simulink model "modele_coque"  (R2025b)
settings: Solver=VariableStepAuto  StartTime=0.0  StopTime=100  RelTol=1e-3
values from neighbouring files (symbols this model uses):
  m = 0.0    (= 0)    [Hulldyn.m]    (also in variables_procom.m = 250000)
  ma = 123434    [variables_procom.m]
  Tc = 0.0    (= 0)    [Hulldyn.m]    (also in variables_procom.m)
settings Model: Creator=leagr  LastModifiedBy=flo

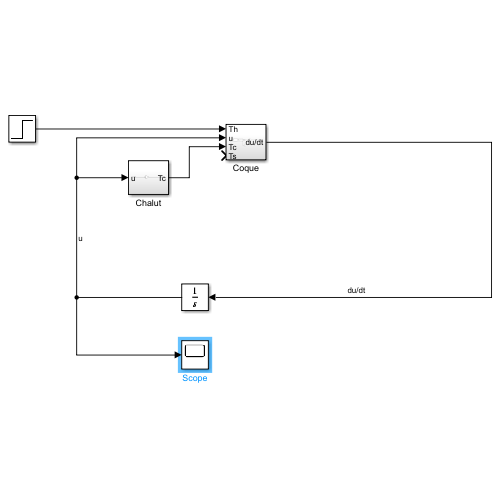
[thumbnail: Simulink's stored preview of the top-level diagram]
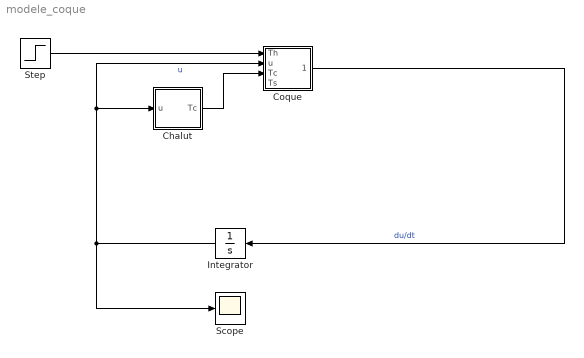
== system modele_coque ==
  Chalut : Subsystem
  Coque : Subsystem
  Integrator : Integrator
  Scope : Scope
      settings: ActiveDisplayYMinimum=-1.0818490746626477  ActiveDisplayYMaximum=9.7366416719638309
  Step : Step  Time=10  After=4e5  SampleTime=0
  wires:
  Coque/1(du/dt) -> Integrator/1  "du/dt"
  Integrator/1 -> Chalut/1(u), Coque/2(u), Scope/1  "u"
  Chalut/1(Tc) -> Coque/3(Tc)
  Step/1 -> Coque/1(Th)

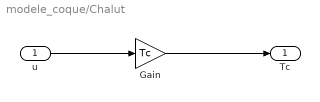
== system modele_coque/Chalut ==
  u : Inport
  Gain : Gain  Gain=Tc
  Tc : Outport
  wires:
  u/1 -> Gain/1
  Gain/1 -> Tc/1

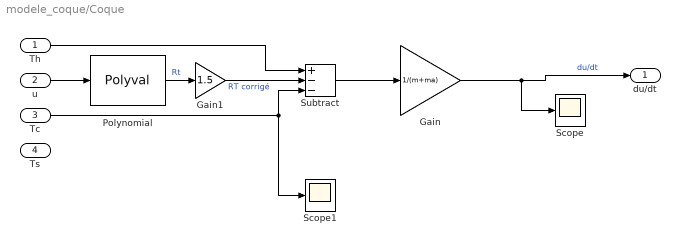
== system modele_coque/Coque ==
  Th : Inport
  u : Inport  Port=2
  Tc : Inport  Port=3
  Ts : Inport  Port=4
  Gain : Gain  Gain=1/(m+ma)
  Gain1 : Gain  Gain=1.5
  Polynomial : Polyval  Coefs=[768.9,-3894,6949.8,-271.6]
  Scope : Scope
      settings: ActiveDisplayYMinimum=-1  ActiveDisplayYMaximum=1
  Scope1 : Scope
      settings: ActiveDisplayYMinimum=-1  ActiveDisplayYMaximum=1  DataLoggingVariableName=ScopeData2
  Subtract : Sum  Inputs=+--
  du/dt : Outport
  wires:
  Subtract/1 -> Gain/1
  Polynomial/1 -> Gain1/1  "Rt"
  Tc/1 -> Scope1/1, Subtract/3
  Gain/1 -> Scope/1, du/dt/1  "du/dt"
  Gain1/1 -> Subtract/2  "RT corrigé"
  u/1 -> Polynomial/1
  Th/1 -> Subtract/1
